simulink model "ContinuousLQG"  (R2015a)
settings: Solver=ode45  StartTime=0.0  StopTime=100  RelTol=1e-3
undefined symbols (not defined in the file): A, B_cont, B_dist, C_sens, Continuous, dt, K_c, SegNum, Time
libraries: ctrlSharedLib x1
settings Model: Creator=Nick  LastModifiedBy=Nick

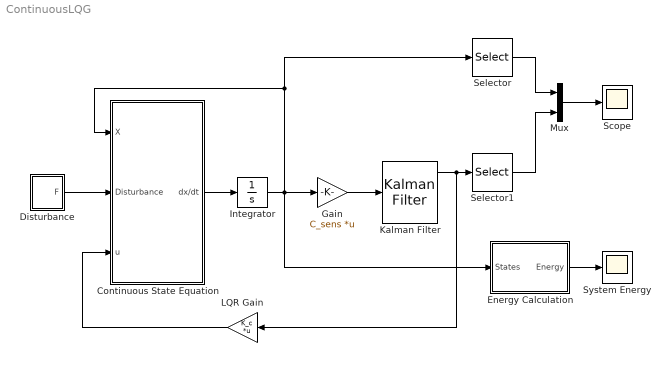
== system ContinuousLQG ==
  Continuous State Equation : Subsystem
  Disturbance : Subsystem
  Energy Calculation : Subsystem
  Gain : Gain  Gain=C_sens  Multiplication=Matrix(K*u)
  Integrator : Integrator
  Kalman Filter : ctrlSharedLib/Kalman Filter  TimeDomain=Continuous-Time  UseCurrentEstimator=on  ModelSource=Individual A, B, C, D matrices  ModelSourceVariable=ss(0.95,1,1,0,1)  A=A  B=B_cont  C=C_sens  D=0  NumberOfStates=1  NumberOfInputs=1  NumberOfOutputs=1  InitialEstimateSource=Dialog  X0=0  P0=10  UseK=off  UseGH=off  NumberOfProcessNoiseInputs=1  G=1  TimeInvariantG=on  H=0  TimeInvariantH=on  Q=10000  TimeInvariantQ=on  R=0.05  TimeInvariantR=on  N=0  TimeInvariantN=on  AddInputPort=off  AddEnablePort=off  ExternalReset=none  OutputEstimatedY=on  OutputP=on  Ts=-1
  LQR Gain : Gain  Gain=K_c  Multiplication=Matrix(K*u)
  Mux : Mux  Inputs=2
  Scope : Scope
      settings: TimeRange=50  YMin=-0.00015  YMax=0.00015
  Selector : Selector  InputPortWidth=length(A)
  Selector1 : Selector  InputPortWidth=length(A)
  System Energy : Scope
      settings: TimeRange=1.742395145364774e-06  YMin=-5.024790181116914e-06  YMax=1.491389349671253e-05  SaveName=StandardEnergy
  wires:
  Disturbance/1(F) -> Continuous State Equation/2(Disturbance)
  Continuous State Equation/1(dx/dt) -> Integrator/1
  Gain/1 -> Kalman Filter/1
  Energy Calculation/1(Energy) -> System Energy/1
  LQR Gain/1 -> Continuous State Equation/3(u)
  Selector/1 -> Mux/1
  Selector1/1 -> Mux/2
  Mux/1 -> Scope/1
  Kalman Filter/1 -> LQR Gain/1, Selector1/1
  Integrator/1 -> Selector/1, Continuous State Equation/1(X), Gain/1, Energy Calculation/1(States)

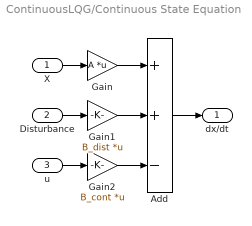
== system ContinuousLQG/Continuous State Equation ==
  X : Inport
  Disturbance : Inport  Port=2
  u : Inport  Port=3
  Add : Sum  Inputs=++-
  Gain : Gain  Gain=A  Multiplication=Matrix(K*u)
  Gain1 : Gain  Gain=B_dist  Multiplication=Matrix(K*u)
  Gain2 : Gain  Gain=B_cont  Multiplication=Matrix(K*u)
  dx/dt : Outport
  wires:
  X/1 -> Gain/1
  Gain/1 -> Add/1
  Disturbance/1 -> Gain1/1
  Gain1/1 -> Add/2
  Add/1 -> dx/dt/1
  u/1 -> Gain2/1
  Gain2/1 -> Add/3

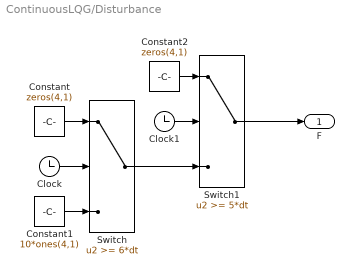
== system ContinuousLQG/Disturbance ==
  Clock : Clock
  Clock1 : Clock
  Constant : Constant  Value=zeros(4,1)
  Constant1 : Constant  Value=10*ones(4,1)
  Constant2 : Constant  Value=zeros(4,1)
  Switch : Switch  Threshold=6*dt
  Switch1 : Switch  Threshold=5*dt
  F : Outport
  wires:
  Clock/1 -> Switch/2
  Constant/1 -> Switch/1
  Constant1/1 -> Switch/3
  Switch/1 -> Switch1/3
  Constant2/1 -> Switch1/1
  Clock1/1 -> Switch1/2
  Switch1/1 -> F/1

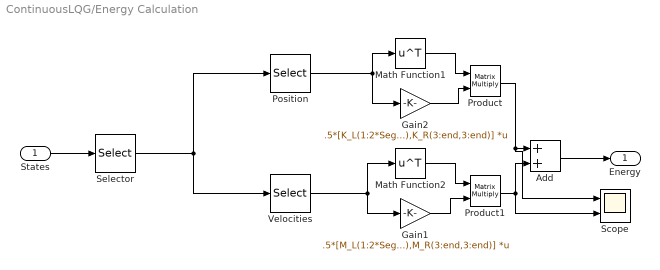
== system ContinuousLQG/Energy Calculation ==
  States : Inport
  Add : Sum
  Gain1 : Gain  Gain=.5*[M_L(1:2*SegNum,1:2*SegNum),zeros(2*SegNum);zeros(2*SegNum),M_R(3:end,3:end)]  Multiplication=Matrix(K*u)
  Gain2 : Gain  Gain=.5*[K_L(1:2*SegNum,1:2*SegNum),zeros(2*SegNum);zeros(2*SegNum),K_R(3:end,3:end)]  Multiplication=Matrix(K*u)
  Math Function1 : Math  Operator=transpose  SaturateOnIntegerOverflow=on
  Math Function2 : Math  Operator=transpose  SaturateOnIntegerOverflow=on
  Position : Selector  InputPortWidth=length(A)-2  Indices=[1:SegNum*4]
  Product : Product  Multiplication=Matrix(*)  RndMeth=Zero
  Product1 : Product  Multiplication=Matrix(*)  RndMeth=Zero
  Scope : Scope  NumInputPorts=2
      settings: YMin=-5~-5  YMax=5~5
  Selector : Selector  InputPortWidth=length(A)  Indices=[1:2*SegNum,2*SegNum+2:6*SegNum+1,6*SegNum+3:length(A)]
  Velocities : Selector  InputPortWidth=length(A)-2  Indices=[SegNum*4+1:SegNum*8]
  Energy : Outport
  wires:
  Position/1 -> Gain2/1, Math Function1/1
  Math Function1/1 -> Product/1
  Gain2/1 -> Product/2
  Velocities/1 -> Gain1/1, Math Function2/1
  Math Function2/1 -> Product1/1
  Gain1/1 -> Product1/2
  Product/1 -> Scope/1, Add/1
  Product1/1 -> Scope/2, Add/2
  Add/1 -> Energy/1
  States/1 -> Selector/1
  Selector/1 -> Position/1, Velocities/1
